simulink model "APTcheck"  (R2021b)
settings: Solver=VariableStepAuto  StartTime=0.0  StopTime=10.0  RelTol=1e-3
settings Model: Creator=Paul  LastModifiedBy=Paul

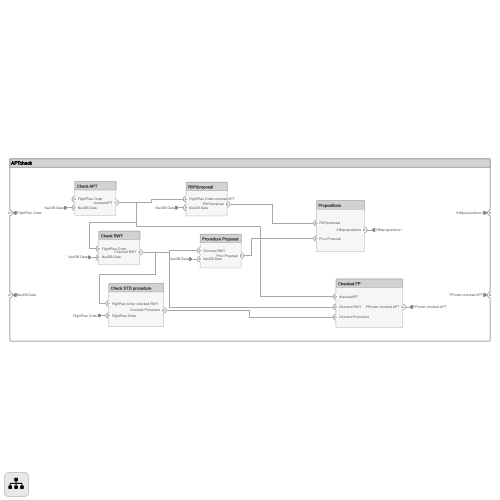
[thumbnail: Simulink's stored preview of the top-level diagram]
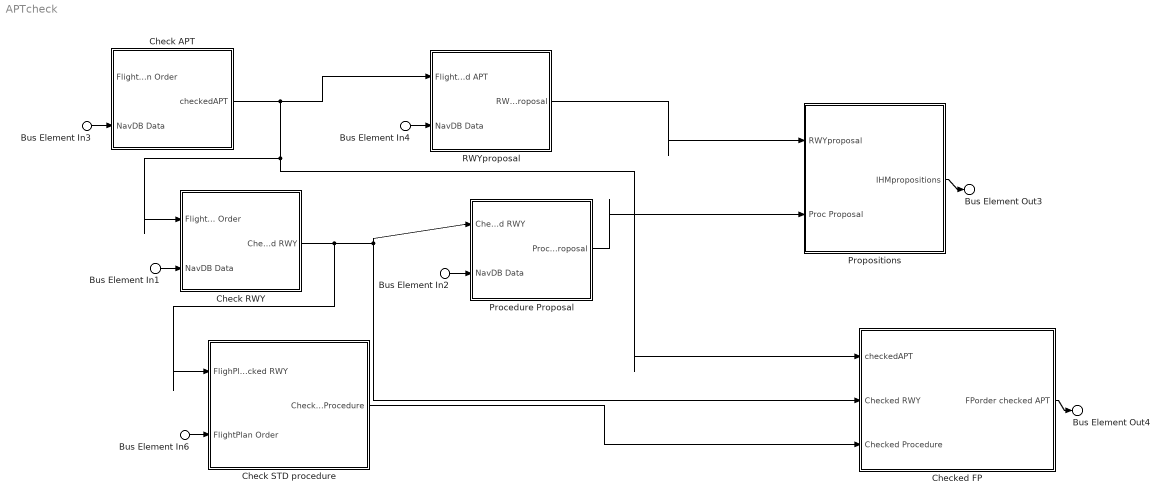
== system APTcheck ==
  Bus Element In6 : Inport  RequirementInfo={} %GIDa_4832b9b0_faf0_49b5_afd4_786529f52d61  PortName=FlightPlan Order
  Bus Element In3 : Inport  RequirementInfo={} %GIDa_f19f8bff_a217_45fa_8fee_83f1e7ee09d3  Port=2  PortName=NavDB Data
  Bus Element In1 : Inport  Port=2  PortName=NavDB Data
  Bus Element In2 : Inport  Port=2  PortName=NavDB Data
  Bus Element In4 : Inport  Port=2  PortName=NavDB Data
  Check APT : Subsystem  RequirementInfo={} %GIDa_cadf43a6_87b2_40b8_978e_fa35865585fd
      settings: PortSchema="{\"entries\":[{\"content\":{\"headerSize\":26,\"margin\":15,\"minimumSpacing\":25,\"sides\":[{\"content\":{\"connectorIds\":[\"In1\",\"In2\"]},\"type\":\"ConnectorPlacement.EquallySpacedRectSide\",\"uuid\":\"3f380961-0284-498f-9d20-a77cf1fdb000\"},{\"content\":{\"connectorIds\":[\"Out1\"],\"side\":\"RIGHT\"},\"type\":\"ConnectorPlacement.EquallySpacedRectSide\",\"uuid\":\"c1cf40f6-b0eb-4111-9692-6c9c6cd53873\"},{\"content\":{\"connectorIds\":[],\"side\":\"TOP\"},\"type\":\"ConnectorPlacement.EquallySpacedRectSide\",\"uuid\":\"4dc1c299-4e42-423b-9cac-e2e11c6bf6b6\"}]},\"type\":\"ConnectorPlacement.EquallySpacedConnector\",\"uuid\":\"af3a7563-dfec-45e0-bdfa-51dd28b27463\"}],\"packageUris\":[\"http://schema.mathworks.com/mf0/Connector/R2020b\"],\"version\":\"1.0\"}"
  Check RWY : Subsystem  RequirementInfo={} %GIDa_145e52e5_61f1_40ee_b829_f8a0c8eeab5e
      settings: PortSchema="{\"entries\":[{\"content\":{\"headerSize\":26,\"margin\":15,\"minimumSpacing\":25,\"sides\":[{\"content\":{\"connectorIds\":[\"In1\",\"In2\"]},\"type\":\"ConnectorPlacement.EquallySpacedRectSide\",\"uuid\":\"3f380961-0284-498f-9d20-a77cf1fdb000\"},{\"content\":{\"connectorIds\":[\"Out1\"],\"side\":\"RIGHT\"},\"type\":\"ConnectorPlacement.EquallySpacedRectSide\",\"uuid\":\"c1cf40f6-b0eb-4111-9692-6c9c6cd53873\"},{\"content\":{\"connectorIds\":[],\"side\":\"TOP\"},\"type\":\"ConnectorPlacement.EquallySpacedRectSide\",\"uuid\":\"4dc1c299-4e42-423b-9cac-e2e11c6bf6b6\"}]},\"type\":\"ConnectorPlacement.EquallySpacedConnector\",\"uuid\":\"af3a7563-dfec-45e0-bdfa-51dd28b27463\"}],\"packageUris\":[\"http://schema.mathworks.com/mf0/Connector/R2020b\"],\"version\":\"1.0\"}"
  Check STD procedure : Subsystem  RequirementInfo={} %GIDa_5a3f482d_31dd_4471_b15f_ba19d595264d
      settings: PortSchema="{\"entries\":[{\"content\":{\"headerSize\":26,\"margin\":15,\"minimumSpacing\":25,\"sides\":[{\"content\":{\"connectorIds\":[\"In1\",\"In2\"]},\"type\":\"ConnectorPlacement.EquallySpacedRectSide\",\"uuid\":\"3f380961-0284-498f-9d20-a77cf1fdb000\"},{\"content\":{\"connectorIds\":[\"Out1\"],\"side\":\"RIGHT\"},\"type\":\"ConnectorPlacement.EquallySpacedRectSide\",\"uuid\":\"c1cf40f6-b0eb-4111-9692-6c9c6cd53873\"},{\"content\":{\"connectorIds\":[],\"side\":\"TOP\"},\"type\":\"ConnectorPlacement.EquallySpacedRectSide\",\"uuid\":\"4dc1c299-4e42-423b-9cac-e2e11c6bf6b6\"}]},\"type\":\"ConnectorPlacement.EquallySpacedConnector\",\"uuid\":\"af3a7563-dfec-45e0-bdfa-51dd28b27463\"}],\"packageUris\":[\"http://schema.mathworks.com/mf0/Connector/R2020b\"],\"version\":\"1.0\"}"
  Checked FP : Subsystem  RequirementInfo={} %GIDa_677b5269_d56e_457e_ac45_3f4a1b06d700
      settings: PortSchema="{\"entries\":[{\"content\":{\"headerSize\":26,\"margin\":15,\"minimumSpacing\":25,\"sides\":[{\"content\":{\"connectorIds\":[\"In1\",\"In2\",\"In3\"]},\"type\":\"ConnectorPlacement.EquallySpacedRectSide\",\"uuid\":\"3f380961-0284-498f-9d20-a77cf1fdb000\"},{\"content\":{\"connectorIds\":[\"Out1\"],\"side\":\"RIGHT\"},\"type\":\"ConnectorPlacement.EquallySpacedRectSide\",\"uuid\":\"c1cf40f6-b0eb-4111-9692-6c9c6cd53873\"},{\"content\":{\"connectorIds\":[],\"side\":\"TOP\"},\"type\":\"ConnectorPlacement.EquallySpacedRectSide\",\"uuid\":\"4dc1c299-4e42-423b-9cac-e2e11c6bf6b6\"}]},\"type\":\"ConnectorPlacement.EquallySpacedConnector\",\"uuid\":\"af3a7563-dfec-45e0-bdfa-51dd28b27463\"}],\"packageUris\":[\"http://schema.mathworks.com/mf0/Connector/R2020b\"],\"version\":\"1.0\"}"
  Procedure Proposal : Subsystem  RequirementInfo={} %GIDa_1a1ec517_75dc_4a0c_81e1_f63806fce986
      settings: PortSchema="{\"entries\":[{\"content\":{\"headerSize\":26,\"margin\":15,\"minimumSpacing\":25,\"sides\":[{\"content\":{\"connectorIds\":[\"In1\",\"In2\"]},\"type\":\"ConnectorPlacement.EquallySpacedRectSide\",\"uuid\":\"3f380961-0284-498f-9d20-a77cf1fdb000\"},{\"content\":{\"connectorIds\":[\"Out1\"],\"side\":\"RIGHT\"},\"type\":\"ConnectorPlacement.EquallySpacedRectSide\",\"uuid\":\"c1cf40f6-b0eb-4111-9692-6c9c6cd53873\"},{\"content\":{\"connectorIds\":[],\"side\":\"TOP\"},\"type\":\"ConnectorPlacement.EquallySpacedRectSide\",\"uuid\":\"4dc1c299-4e42-423b-9cac-e2e11c6bf6b6\"}]},\"type\":\"ConnectorPlacement.EquallySpacedConnector\",\"uuid\":\"af3a7563-dfec-45e0-bdfa-51dd28b27463\"}],\"packageUris\":[\"http://schema.mathworks.com/mf0/Connector/R2020b\"],\"version\":\"1.0\"}"
  Propositions : Subsystem  RequirementInfo={} %GIDa_3d39a334_d73d_4c5a_8005_74029ba4b4be
      settings: PortSchema="{\"entries\":[{\"content\":{\"headerSize\":26,\"margin\":15,\"minimumSpacing\":25,\"sides\":[{\"content\":{\"connectorIds\":[\"In1\",\"In2\"]},\"type\":\"ConnectorPlacement.EquallySpacedRectSide\",\"uuid\":\"3f380961-0284-498f-9d20-a77cf1fdb000\"},{\"content\":{\"connectorIds\":[\"Out1\"],\"side\":\"RIGHT\"},\"type\":\"ConnectorPlacement.EquallySpacedRectSide\",\"uuid\":\"c1cf40f6-b0eb-4111-9692-6c9c6cd53873\"},{\"content\":{\"connectorIds\":[],\"side\":\"TOP\"},\"type\":\"ConnectorPlacement.EquallySpacedRectSide\",\"uuid\":\"4dc1c299-4e42-423b-9cac-e2e11c6bf6b6\"}]},\"type\":\"ConnectorPlacement.EquallySpacedConnector\",\"uuid\":\"af3a7563-dfec-45e0-bdfa-51dd28b27463\"}],\"packageUris\":[\"http://schema.mathworks.com/mf0/Connector/R2020b\"],\"version\":\"1.0\"}"
  RWYproposal : Subsystem  RequirementInfo={} %GIDa_8b4bf1da_c5c9_4940_906d_45790737c397
      settings: PortSchema="{\"entries\":[{\"content\":{\"headerSize\":26,\"margin\":15,\"minimumSpacing\":25,\"sides\":[{\"content\":{\"connectorIds\":[\"In1\",\"In2\"]},\"type\":\"ConnectorPlacement.EquallySpacedRectSide\",\"uuid\":\"3f380961-0284-498f-9d20-a77cf1fdb000\"},{\"content\":{\"connectorIds\":[\"Out1\"],\"side\":\"RIGHT\"},\"type\":\"ConnectorPlacement.EquallySpacedRectSide\",\"uuid\":\"c1cf40f6-b0eb-4111-9692-6c9c6cd53873\"},{\"content\":{\"connectorIds\":[],\"side\":\"TOP\"},\"type\":\"ConnectorPlacement.EquallySpacedRectSide\",\"uuid\":\"4dc1c299-4e42-423b-9cac-e2e11c6bf6b6\"}]},\"type\":\"ConnectorPlacement.EquallySpacedConnector\",\"uuid\":\"af3a7563-dfec-45e0-bdfa-51dd28b27463\"}],\"packageUris\":[\"http://schema.mathworks.com/mf0/Connector/R2020b\"],\"version\":\"1.0\"}"
  Bus Element Out3 : Outport  RequirementInfo={} %GIDa_80b212ac_695d_483d_be3a_9a78cd1f5e7d  PortName=IHMpropositions
  Bus Element Out4 : Outport  RequirementInfo={} %GIDa_10d13ba6_314e_4501_951d_9b0539b57921  Port=2  PortName=FPorder checked APT
  wires:
  Check RWY/1(Checked RWY) -> Checked FP/2(Checked RWY), Procedure Proposal/1(Checked RWY), Check STD procedure/1(FlighPlan Order checked RWY)
  Bus Element In6/1 -> Check STD procedure/2(FlightPlan Order)
  Check STD procedure/1(Checked Procedure) -> Checked FP/3(Checked Procedure)
  Bus Element In1/1 -> Check RWY/2(NavDB Data)
  Bus Element In4/1 -> RWYproposal/2(NavDB Data)
  Check APT/1(checkedAPT) -> RWYproposal/1(FlightPlan Order checked APT), Checked FP/1(checkedAPT), Check RWY/1(FlightPlan Order)
  Propositions/1(IHMpropositions) -> Bus Element Out3/1
  RWYproposal/1(RWYproposal) -> Propositions/1(RWYproposal)
  Bus Element In3/1 -> Check APT/2(NavDB Data)
  Bus Element In2/1 -> Procedure Proposal/2(NavDB Data)
  Procedure Proposal/1(Proc Proposal) -> Propositions/2(Proc Proposal)
  Checked FP/1(FPorder checked APT) -> Bus Element Out4/1

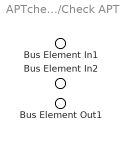
== system APTcheck/Check APT ==
  Bus Element In1 : Inport  RequirementInfo={} %GIDa_9eb3bd42_df3e_447a_9e89_fbb7e1664a7e  PortName=FlightPlan Order
  Bus Element In2 : Inport  RequirementInfo={} %GIDa_f89291ea_421b_46b8_a44d_82d29a48bf13  Port=2  PortName=NavDB Data
  Bus Element Out1 : Outport  RequirementInfo={} %GIDa_45e647ad_242e_4185_8771_2f174731fe89  PortName=checkedAPT

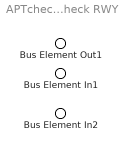
== system APTcheck/Check RWY ==
  Bus Element In1 : Inport  RequirementInfo={} %GIDa_1e4df057_0859_4e77_9408_6349eb4848a2  PortName=FlightPlan Order
  Bus Element In2 : Inport  RequirementInfo={} %GIDa_b0c658e9_4791_4149_83e1_35dd945bd6d8  Port=2  PortName=NavDB Data
  Bus Element Out1 : Outport  RequirementInfo={} %GIDa_144afadf_3cfa_4b43_b3cf_0c66b8a546d1  PortName=Checked RWY

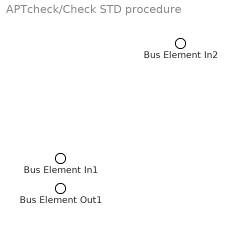
== system APTcheck/Check STD procedure ==
  Bus Element In2 : Inport  RequirementInfo={} %GIDa_63e91bc5_1537_4067_8ecd_c2e49a42424d  PortName=FlighPlan Order checked RWY
  Bus Element In1 : Inport  RequirementInfo={} %GIDa_cbb80570_74c6_4e04_bd0f_357178818488  Port=2  PortName=FlightPlan Order
  Bus Element Out1 : Outport  RequirementInfo={} %GIDa_f1f01310_eb8a_4d64_b369_59fe6a984d21  PortName=Checked Procedure

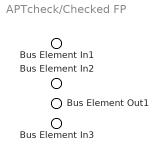
== system APTcheck/Checked FP ==
  Bus Element In1 : Inport  RequirementInfo={} %GIDa_a694f201_b6cc_4e59_a602_245e49348ff2  PortName=checkedAPT
  Bus Element In2 : Inport  RequirementInfo={} %GIDa_a90aca41_2af9_462a_b36a_268b96c48eac  Port=2  PortName=Checked RWY
  Bus Element In3 : Inport  RequirementInfo={} %GIDa_e6311af9_d7d3_4295_86f3_87d4a9b5275d  Port=3  PortName=Checked Procedure
  Bus Element Out1 : Outport  RequirementInfo={} %GIDa_fbf3b13c_df8c_4670_8c18_a1798f0c1edd  PortName=FPorder checked APT

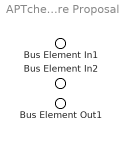
== system APTcheck/Procedure Proposal ==
  Bus Element In1 : Inport  RequirementInfo={} %GIDa_6b03d257_6c93_447d_9d99_f174614d021a  PortName=Checked RWY
  Bus Element In2 : Inport  RequirementInfo={} %GIDa_65230ea7_7ef1_45b1_a67b_c7b33448d676  Port=2  PortName=NavDB Data
  Bus Element Out1 : Outport  RequirementInfo={} %GIDa_d794938f_0d1b_4b31_949a_ee55ae9a7a39  PortName=Proc Proposal

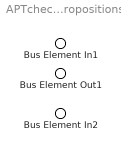
== system APTcheck/Propositions ==
  Bus Element In1 : Inport  RequirementInfo={} %GIDa_08b4c3a0_8b2e_4945_8454_29d4f031e2e1  PortName=RWYproposal
  Bus Element In2 : Inport  RequirementInfo={} %GIDa_dfa5f984_86f3_4a75_aa99_c9cf09258d5c  Port=2  PortName=Proc Proposal
  Bus Element Out1 : Outport  RequirementInfo={} %GIDa_0fc6203a_1287_43ba_87dd_e2105230476b  PortName=IHMpropositions

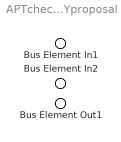
== system APTcheck/RWYproposal ==
  Bus Element In1 : Inport  RequirementInfo={} %GIDa_d175aadf_2d94_4bc9_9cd2_2e5f93ec3a8c  PortName=FlightPlan Order checked APT
  Bus Element In2 : Inport  RequirementInfo={} %GIDa_45022dca_7b90_4a9f_9039_a5d6aea7fba1  Port=2  PortName=NavDB Data
  Bus Element Out1 : Outport  RequirementInfo={} %GIDa_c9a6e321_2c59_4b3d_be25_a490cff97f7f  PortName=RWYproposal
